simulink model "TDMA_mao"  (R2016a)
settings: Solver=VariableStepAuto  StartTime=0.0  StopTime=10.0  RelTol=1e-3
libraries: commrandsrc3 x4, commsink2 x4, commrflib2 x2, commdigbbndpm3 x2
settings Model: Creator=Mao Jianqiao  LastModifiedBy=Mao Jianqiao

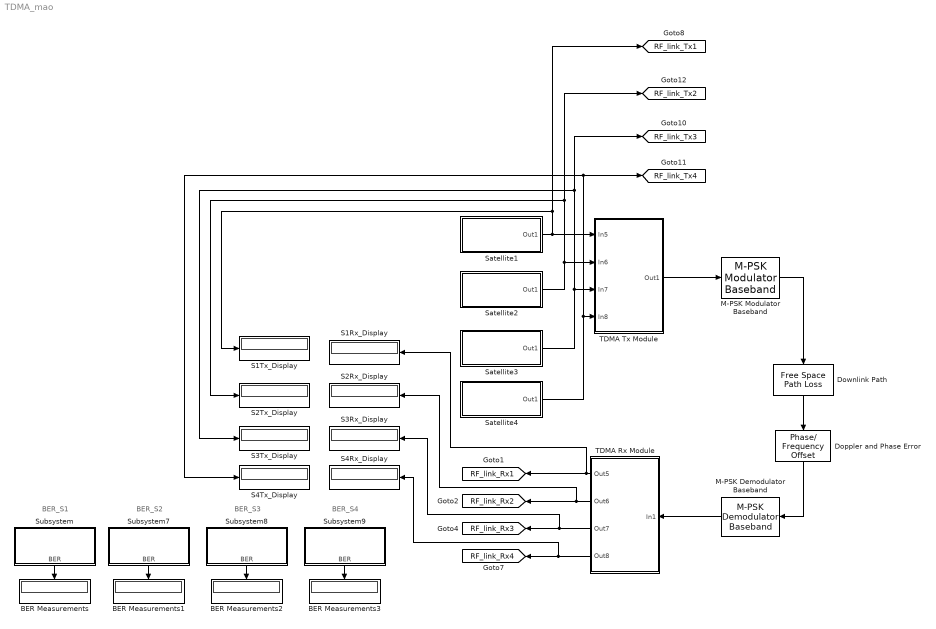
== system TDMA_mao ==
  note: BER_S1
  note: BER_S2
  note: BER_S3
  note: BER_S4
  BER Measurements{,1..3} (4 alike) : Display
      settings: Format=short_e
  Doppler and Phase Error : commrflib2/Phase// Frequency Offset  phaseOffset=0  freqPort=off  freqOffset=paramRFSatLink.DoppOffset
  Downlink Path : commrflib2/Free Space Path Loss  mode=Distance and Frequency  dB=180  d=paramRFSatLink.Altitude  fc=paramRFSatLink.Frequency
  M-PSK Demodulator Baseband : commdigbbndpm3/M-PSK Demodulator Baseband  M=8  OutType=Integer  DecType=Hard decision  VarSource=Dialog  Variance=1  Dec=Gray  Mapping=[0:7]  Ph=pi/8  outDtype1=Inherit via internal rule  outDtype2=Inherit via internal rule  derotateFactorWordLen=16  derotateFactorDataTypeStr=Inherit: Same word length as input  derotateFactorLastDataTypeStr=Inherit: Same word length as input
  M-PSK Modulator Baseband : commdigbbndpm3/M-PSK Modulator Baseband  M=8  InType=Integer  Enc=Gray  Mapping=[0:7]  Ph=pi/8  outDtype=double  outWordLen=16  outUDDataType=sfix(16)  outFracLenMode=Best precision  outFracLen=15  outDataTypeStr=double  outLastDataTypeStr=double
  S1Rx_Display : Display
  S1Tx_Display : Display
  S2Rx_Display : Display
  S2Tx_Display : Display
  S3Rx_Display : Display
  S3Tx_Display : Display
  S4Rx_Display : Display
  S4Tx_Display : Display
  Satellite1 : Subsystem
  Satellite2 : Subsystem
  Satellite3 : Subsystem
  Satellite4 : Subsystem
  Subsystem : Subsystem
      mask Display: disp('Display Complete\nBit Error Rate\nInformation');
  Subsystem7 : Subsystem
      mask Display: disp('Display Complete\nBit Error Rate\nInformation');
  Subsystem8 : Subsystem
      mask Display: disp('Display Complete\nBit Error Rate\nInformation');
  Subsystem9 : Subsystem
      mask Display: disp('Display Complete\nBit Error Rate\nInformation');
  TDMA Rx Module : Subsystem
  TDMA Tx Module : Subsystem
  tag scope: RF_link_Rx1=global, RF_link_Rx2=global, RF_link_Rx3=global, RF_link_Rx4=global, RF_link_Tx1=global, RF_link_Tx2=global, RF_link_Tx3=global, RF_link_Tx4=global
  wires:
  TDMA Rx Module/1(Out5) -> S1Rx_Display/1, [RF_link_Rx1]
  TDMA Rx Module/2(Out6) -> S2Rx_Display/1, [RF_link_Rx2]
  TDMA Rx Module/3(Out7) -> S3Rx_Display/1, [RF_link_Rx3]
  TDMA Rx Module/4(Out8) -> S4Rx_Display/1, [RF_link_Rx4]
  Satellite1/1(Out1) -> [RF_link_Tx1], S1Tx_Display/1, TDMA Tx Module/1(In5)
  Satellite2/1(Out1) -> [RF_link_Tx2], S2Tx_Display/1, TDMA Tx Module/2(In6)
  Satellite3/1(Out1) -> TDMA Tx Module/3(In7), [RF_link_Tx3], S3Tx_Display/1
  Satellite4/1(Out1) -> S4Tx_Display/1, [RF_link_Tx4], TDMA Tx Module/4(In8)
  Subsystem/1(BER) -> BER Measurements/1
  Subsystem7/1(BER) -> BER Measurements1/1
  Subsystem8/1(BER) -> BER Measurements2/1
  Subsystem9/1(BER) -> BER Measurements3/1
  TDMA Tx Module/1(Out1) -> M-PSK Modulator Baseband/1
  M-PSK Modulator Baseband/1 -> Downlink Path/1
  M-PSK Demodulator Baseband/1 -> TDMA Rx Module/1(In1)
  Downlink Path/1 -> Doppler and Phase Error/1
  Doppler and Phase Error/1 -> M-PSK Demodulator Baseband/1

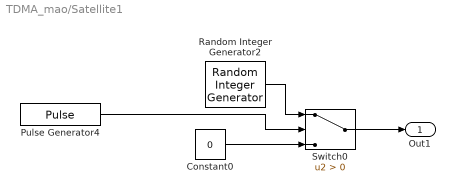
== system TDMA_mao/Satellite1 ==
  Constant0 : Constant  Value=0
  Pulse Generator4 : DiscretePulseGenerator  Period=4  SampleTime=1/10000000
  Random Integer Generator2 : commrandsrc3/Random Integer Generator  SetSize=8  SeedSource=Parameter  Seed=13  SampleTime=1/10000000  SamplesPerFrame=1  OutputDataType=double  SimulateUsing=Interpreted execution
  Switch0 : Switch  Criteria=u2 > Threshold
  Out1 : Outport
  wires:
  Random Integer Generator2/1 -> Switch0/1
  Pulse Generator4/1 -> Switch0/2
  Constant0/1 -> Switch0/3
  Switch0/1 -> Out1/1

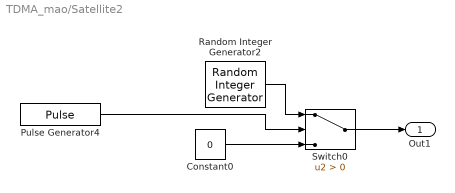
== system TDMA_mao/Satellite2 ==
  Constant0 : Constant  Value=0
  Pulse Generator4 : DiscretePulseGenerator  Period=4  PhaseDelay=1  SampleTime=1/10000000
  Random Integer Generator2 : commrandsrc3/Random Integer Generator  SetSize=8  SeedSource=Parameter  Seed=13  SampleTime=1/10000000  SamplesPerFrame=1  OutputDataType=double  SimulateUsing=Interpreted execution
  Switch0 : Switch  Criteria=u2 > Threshold
  Out1 : Outport
  wires:
  Random Integer Generator2/1 -> Switch0/1
  Pulse Generator4/1 -> Switch0/2
  Constant0/1 -> Switch0/3
  Switch0/1 -> Out1/1

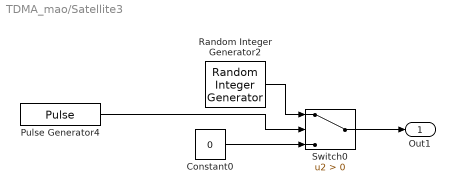
== system TDMA_mao/Satellite3 ==
  Constant0 : Constant  Value=0
  Pulse Generator4 : DiscretePulseGenerator  Period=4  PhaseDelay=2  SampleTime=1/10000000
  Random Integer Generator2 : commrandsrc3/Random Integer Generator  SetSize=8  SeedSource=Parameter  Seed=13  SampleTime=1/10000000  SamplesPerFrame=1  OutputDataType=double  SimulateUsing=Interpreted execution
  Switch0 : Switch  Criteria=u2 > Threshold
  Out1 : Outport
  wires:
  Random Integer Generator2/1 -> Switch0/1
  Pulse Generator4/1 -> Switch0/2
  Constant0/1 -> Switch0/3
  Switch0/1 -> Out1/1

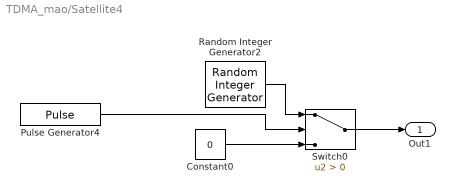
== system TDMA_mao/Satellite4 ==
  Constant0 : Constant  Value=0
  Pulse Generator4 : DiscretePulseGenerator  Period=4  PhaseDelay=3  SampleTime=1/10000000
  Random Integer Generator2 : commrandsrc3/Random Integer Generator  SetSize=8  SeedSource=Parameter  Seed=13  SampleTime=1/10000000  SamplesPerFrame=1  OutputDataType=double  SimulateUsing=Interpreted execution
  Switch0 : Switch  Criteria=u2 > Threshold
  Out1 : Outport
  wires:
  Random Integer Generator2/1 -> Switch0/1
  Pulse Generator4/1 -> Switch0/2
  Constant0/1 -> Switch0/3
  Switch0/1 -> Out1/1

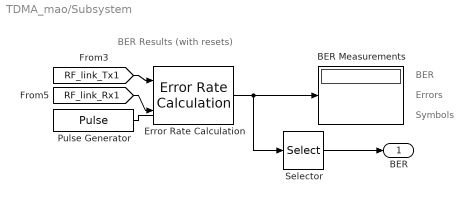
== system TDMA_mao/Subsystem ==
  note: BER
  note: Errors
  note: Symbols
  note: BER Results (with resets)
  BER Measurements : Display
  Error Rate Calculation : commsink2/Error Rate Calculation  N=0  st_delay=0  cp_mode=Entire frame  subframe=[]  PMode=Port  WsName=ErrorVec  RsMode2=off  stop=off  numErr=200  maxBits=1e6
  Pulse Generator : DiscretePulseGenerator  Period=100  SampleTime=1/10000000
  Selector : Selector  InputPortWidth=3  IndexOptions=Index vector (dialog)  Indices=[1]  OutputSizes=1
  BER : Outport
  wires:
  [RF_link_Tx1] -> Error Rate Calculation/1
  [RF_link_Rx1] -> Error Rate Calculation/2
  Error Rate Calculation/1 -> BER Measurements/1, Selector/1
  Pulse Generator/1 -> ?
  Selector/1 -> BER/1

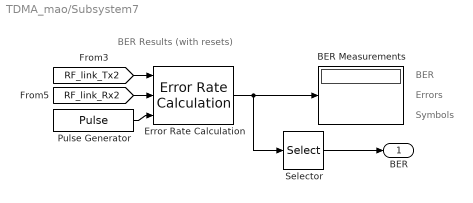
== system TDMA_mao/Subsystem7 ==
  note: BER
  note: Errors
  note: Symbols
  note: BER Results (with resets)
  BER Measurements : Display
  Error Rate Calculation : commsink2/Error Rate Calculation  N=0  st_delay=0  cp_mode=Entire frame  subframe=[]  PMode=Port  WsName=ErrorVec  RsMode2=on  stop=off  numErr=200  maxBits=1e6
  Pulse Generator : DiscretePulseGenerator  Period=100  SampleTime=1/10000000
  Selector : Selector  InputPortWidth=3  IndexOptions=Index vector (dialog)  Indices=[1]  OutputSizes=1
  BER : Outport
  wires:
  [RF_link_Tx2] -> Error Rate Calculation/1
  [RF_link_Rx2] -> Error Rate Calculation/2
  Error Rate Calculation/1 -> BER Measurements/1, Selector/1
  Pulse Generator/1 -> Error Rate Calculation/3
  Selector/1 -> BER/1

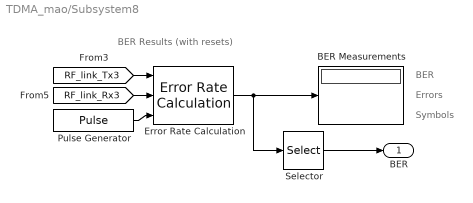
== system TDMA_mao/Subsystem8 ==
  note: BER
  note: Errors
  note: Symbols
  note: BER Results (with resets)
  BER Measurements : Display
  Error Rate Calculation : commsink2/Error Rate Calculation  N=0  st_delay=0  cp_mode=Entire frame  subframe=[]  PMode=Port  WsName=ErrorVec  RsMode2=on  stop=off  numErr=200  maxBits=1e6
  Pulse Generator : DiscretePulseGenerator  Period=100  SampleTime=1/10000000
  Selector : Selector  InputPortWidth=3  IndexOptions=Index vector (dialog)  Indices=[1]  OutputSizes=1
  BER : Outport
  wires:
  [RF_link_Tx3] -> Error Rate Calculation/1
  [RF_link_Rx3] -> Error Rate Calculation/2
  Error Rate Calculation/1 -> BER Measurements/1, Selector/1
  Pulse Generator/1 -> Error Rate Calculation/3
  Selector/1 -> BER/1

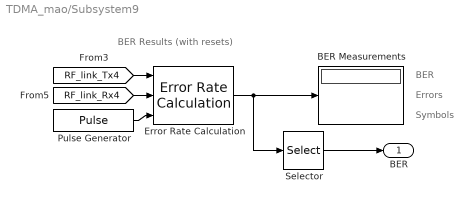
== system TDMA_mao/Subsystem9 ==
  note: BER
  note: Errors
  note: Symbols
  note: BER Results (with resets)
  BER Measurements : Display
  Error Rate Calculation : commsink2/Error Rate Calculation  N=0  st_delay=0  cp_mode=Entire frame  subframe=[]  PMode=Port  WsName=ErrorVec  RsMode2=on  stop=off  numErr=200  maxBits=1e6
  Pulse Generator : DiscretePulseGenerator  Period=100  SampleTime=1/10000000
  Selector : Selector  InputPortWidth=3  IndexOptions=Index vector (dialog)  Indices=[1]  OutputSizes=1
  BER : Outport
  wires:
  [RF_link_Tx4] -> Error Rate Calculation/1
  [RF_link_Rx4] -> Error Rate Calculation/2
  Error Rate Calculation/1 -> BER Measurements/1, Selector/1
  Pulse Generator/1 -> Error Rate Calculation/3
  Selector/1 -> BER/1

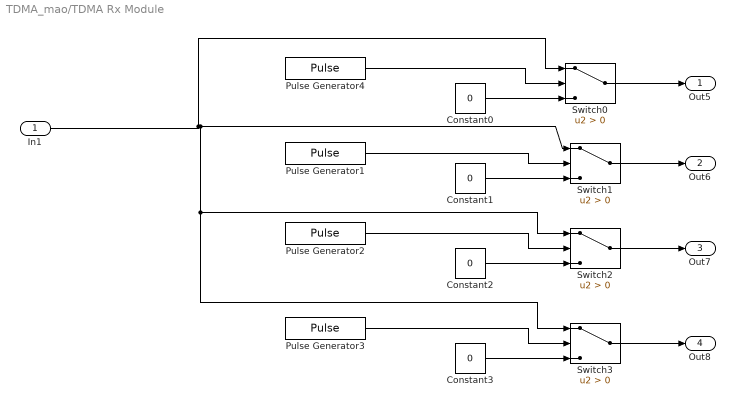
== system TDMA_mao/TDMA Rx Module ==
  In1 : Inport
  Constant{0..3} (4 alike) : Constant  Value=0
  Pulse Generator1 : DiscretePulseGenerator  Period=4  PhaseDelay=1  SampleTime=1/10000000
  Pulse Generator2 : DiscretePulseGenerator  Period=4  PhaseDelay=2  SampleTime=1/10000000
  Pulse Generator3 : DiscretePulseGenerator  Period=4  PhaseDelay=3  SampleTime=1/10000000
  Pulse Generator4 : DiscretePulseGenerator  Period=4  SampleTime=1/10000000
  Switch{0..3} (4 alike) : Switch  Criteria=u2 > Threshold
  Out5 : Outport
  Out6 : Outport  Port=2
  Out7 : Outport  Port=3
  Out8 : Outport  Port=4
  wires:
  Constant2/1 -> Switch2/3
  Constant1/1 -> Switch1/3
  Constant0/1 -> Switch0/3
  Pulse Generator1/1 -> Switch1/2
  Pulse Generator4/1 -> Switch0/2
  Pulse Generator2/1 -> Switch2/2
  Switch0/1 -> Out5/1
  Switch2/1 -> Out7/1
  Switch1/1 -> Out6/1
  Constant3/1 -> Switch3/3
  Pulse Generator3/1 -> Switch3/2
  In1/1 -> Switch0/1, Switch3/1, Switch2/1, Switch1/1
  Switch3/1 -> Out8/1

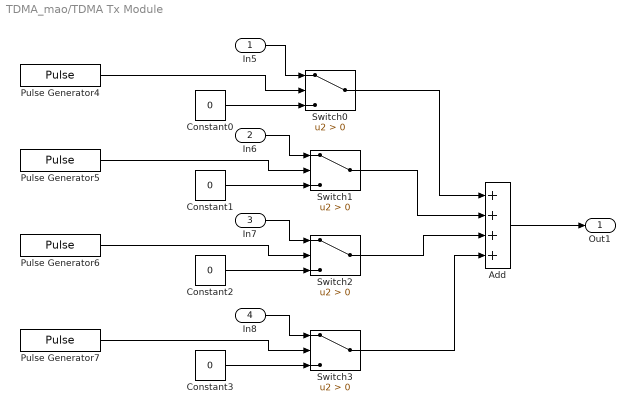
== system TDMA_mao/TDMA Tx Module ==
  In5 : Inport
  In6 : Inport  Port=2
  In7 : Inport  Port=3
  In8 : Inport  Port=4
  Add : Sum  Inputs=++++
  Constant{0..3} (4 alike) : Constant  Value=0
  Pulse Generator4 : DiscretePulseGenerator  Period=4  SampleTime=1/10000000
  Pulse Generator5 : DiscretePulseGenerator  Period=4  PhaseDelay=1  SampleTime=1/10000000
  Pulse Generator6 : DiscretePulseGenerator  Period=4  PhaseDelay=2  SampleTime=1/10000000
  Pulse Generator7 : DiscretePulseGenerator  Period=4  PhaseDelay=3  SampleTime=1/10000000
  Switch{0..3} (4 alike) : Switch  Criteria=u2 > Threshold
  Out1 : Outport
  wires:
  Add/1 -> Out1/1
  Switch3/1 -> Add/4
  In8/1 -> Switch3/1
  Pulse Generator7/1 -> Switch3/2
  Constant3/1 -> Switch3/3
  Switch1/1 -> Add/2
  Switch2/1 -> Add/3
  Switch0/1 -> Add/1
  In7/1 -> Switch2/1
  In6/1 -> Switch1/1
  In5/1 -> Switch0/1
  Pulse Generator6/1 -> Switch2/2
  Pulse Generator4/1 -> Switch0/2
  Pulse Generator5/1 -> Switch1/2
  Constant0/1 -> Switch0/3
  Constant1/1 -> Switch1/3
  Constant2/1 -> Switch2/3
